simulink model "hpt_1to1_switchlevel"  (R2025a)
settings: Solver=ode23tb  StartTime=0.0  StopTime=0.02  RelTol=1e-3
libraries: spsIGBTLib x19, spsLinearTransformerLib x9, spsGroundLib x4, spsThreePhaseVIMeasurementLib x3, spsSeriesRLCBranchLib x2, spsThreePhaseSeriesRLCBranchLib x2, spsThreePhaseSourceLib x1, spsThreePhaseSeriesRLCLoadLib x1, spsVoltageMeasurementLib x1, spspowerguiLib x1
settings Model: Creator=m1391  LastModifiedBy=m1391

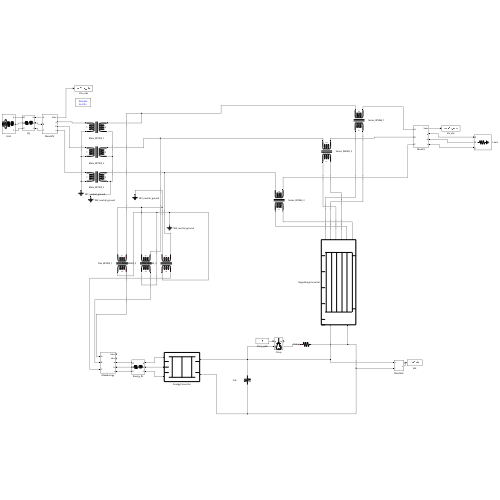
[thumbnail: Simulink's stored preview of the top-level diagram]
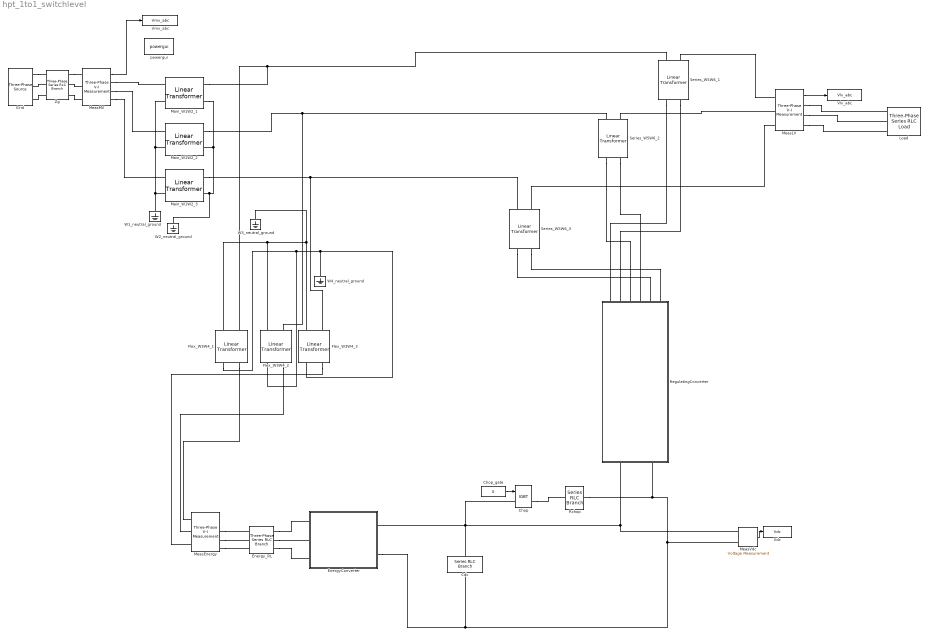
== system hpt_1to1_switchlevel ==
  Cdc : spsSeriesRLCBranchLib/Series RLC Branch  LConnTagsString=__new0  RConnTagsString=__new0  BranchType=C  Resistance=1  Inductance=1e-3  SetiL0=off  InitialCurrent=0  Capacitance=0.0022  Setx0=on  InitialVoltage=800  Measurements=None
  Chop : spsIGBTLib/IGBT  Ron=0.001  Lon=0  Vf=1  Tf=1e-6  Tt=2e-6  IC=0  Rs=1e5  Cs=inf  Measurements=on
  Chop_gate : Constant  Value=0
  EnergyConverter : Subsystem
      mask Display:
      | color('black');
      | plot([10 90 90 10 10],[10 10 90 90 10]);
      | plot([20 80],[78 78]); plot([20 80],[22 22]);
      | plot([28 28],[22 78]); plot([50 50],[22 78]); plot([72 72],[22 78]);
      | plot([10 20],[65 65]); plot([10 20],[50 50]); plot([10 20],[35 35]);
      | plot([80 90],[65 65]); plot([80 90],[35 35]);
  Energy_RL : spsThreePhaseSeriesRLCBranchLib/Three-Phase Series RLC Branch  LConnTagsString=A|B|C  RConnTagsString=A|B|C  BranchType=RL  Resistance=0.05  Inductance=0.003  Capacitance=1e-6  Measurements=None
  Flex_W3W4_1 : spsLinearTransformerLib/Linear Transformer  UNITS=pu  NominalPower=[40000,50]  winding1=[230.9401,0.005,0.02]  winding2=[230.9401,0.005,0.02]  ThreeWindings=off  winding3=[ 315e3 0.002 0.08 ]  RmLm=[ 500 500 ]  Measurements=None  DataType=off
  Flex_W3W4_2 : spsLinearTransformerLib/Linear Transformer  UNITS=pu  NominalPower=[40000,50]  winding1=[230.9401,0.005,0.02]  winding2=[230.9401,0.005,0.02]  ThreeWindings=off  winding3=[ 315e3 0.002 0.08 ]  RmLm=[ 500 500 ]  Measurements=None  DataType=off
  Flex_W3W4_3 : spsLinearTransformerLib/Linear Transformer  UNITS=pu  NominalPower=[40000,50]  winding1=[230.9401,0.005,0.02]  winding2=[230.9401,0.005,0.02]  ThreeWindings=off  winding3=[ 315e3 0.002 0.08 ]  RmLm=[ 500 500 ]  Measurements=None  DataType=off
  Grid : spsThreePhaseSourceLib/Three-Phase Source  InternalConnection=Yg  VoltagePhases=off  Voltage=10000  PhaseAngle=0  Voltage_phases=[25e3 25e3 25e3]/sqrt(3)  PhaseAngles_phases=[0 -120 +120]  Frequency=50  NonIdealSource=on  SpecifyImpedance=off  Resistance=1e-3  Inductance=1e-5  ShortCircuitLevel=100e6  BaseVoltage=25e3  XRratio=7  BusType=swing  Pref=10e3  Qref=0  Prefabc=[10e3, 10e3, 10e3]  Qrefabc=[0, 0, 0]  Qmin=-inf  Qmax=inf
  Load : spsThreePhaseSeriesRLCLoadLib/Three-Phase Series RLC Load  LConnTagsString=A|B|C  Configuration=Y (grounded)  NominalVoltage=400  Vabc=[1e3 1e3 1e3]  Vabcp=[1e3 1e3 1e3]  NominalFrequency=50  UnbalancedPower=off  ActivePower=400000  InductivePower=0  CapacitivePower=0  Pabc=[10e3 9e3 11e3]  QLabc=[100 90 110]  QCabc=[100 90 110]  Pabcp=[10e3 9e3 11e3]  QLabcp=[100 90 110]  QCabcp=[100 90 110]  Measurements=None  LoadType=constant Z
  Main_W1W2_1 : spsLinearTransformerLib/Linear Transformer  UNITS=pu  NominalPower=[133333.3333,50]  winding1=[5773.5027,0.005,0.025]  winding2=[230.9401,0.005,0.025]  ThreeWindings=off  winding3=[ 315e3 0.002 0.08 ]  RmLm=[ 500 500 ]  Measurements=None  DataType=off
  Main_W1W2_2 : spsLinearTransformerLib/Linear Transformer  UNITS=pu  NominalPower=[133333.3333,50]  winding1=[5773.5027,0.005,0.025]  winding2=[230.9401,0.005,0.025]  ThreeWindings=off  winding3=[ 315e3 0.002 0.08 ]  RmLm=[ 500 500 ]  Measurements=None  DataType=off
  Main_W1W2_3 : spsLinearTransformerLib/Linear Transformer  UNITS=pu  NominalPower=[133333.3333,50]  winding1=[5773.5027,0.005,0.025]  winding2=[230.9401,0.005,0.025]  ThreeWindings=off  winding3=[ 315e3 0.002 0.08 ]  RmLm=[ 500 500 ]  Measurements=None  DataType=off
  MeasEnergy : spsThreePhaseVIMeasurementLib/Three-Phase V-I Measurement  VoltageMeasurement=phase-to-ground  SetLabelV=off  LabelV=Vabc  Vpu=off  VpuLL=off  CurrentMeasurement=yes  SetLabelI=off  LabelI=Iabc  Ipu=off  Pbase=100e6  Vbase=500e3  OutputType=Complex  PhasorSimulation=off  PSBequivalent=0
  MeasLV : spsThreePhaseVIMeasurementLib/Three-Phase V-I Measurement  VoltageMeasurement=phase-to-ground  SetLabelV=off  LabelV=Vabc  Vpu=off  VpuLL=off  CurrentMeasurement=no  SetLabelI=off  LabelI=Iabc  Ipu=off  Pbase=100e6  Vbase=500e3  OutputType=Complex  PhasorSimulation=off  PSBequivalent=0
  MeasMV : spsThreePhaseVIMeasurementLib/Three-Phase V-I Measurement  VoltageMeasurement=phase-to-ground  SetLabelV=off  LabelV=Vabc  Vpu=off  VpuLL=off  CurrentMeasurement=no  SetLabelI=off  LabelI=Iabc  Ipu=off  Pbase=100e6  Vbase=500e3  OutputType=Complex  PhasorSimulation=off  PSBequivalent=0
  MeasVdc : spsVoltageMeasurementLib/Voltage Measurement  PhasorSimulation=off  OutputType=Complex  PSBequivalent=0
  Rchop : spsSeriesRLCBranchLib/Series RLC Branch  LConnTagsString=__new0  RConnTagsString=__new0  BranchType=R  Resistance=5.3333  Inductance=1e-3  SetiL0=off  InitialCurrent=0  Capacitance=1e-6  Setx0=off  InitialVoltage=0  Measurements=None
  RegulatingConverter : Subsystem
      mask Display:
      | color('black');
      | plot([5 95 95 5 5],[10 10 90 90 10]);
      | plot([15 85],[78 78]); plot([15 85],[22 22]);
      | plot([18 18],[22 78]); plot([32 32],[22 78]);
      | plot([45 45],[22 78]); plot([59 59],[22 78]);
      | plot([72 72],[22 78]); plot([86 86],[22 78]);
      | plot([5 15],[75 75]); plot([5 15],[60 60]); plot([5 15],[45 45]);
      | plot([5 15],[30 30]); plot([5 15],[15 15]); plot([5 15],[10 10]);
      | plot([85 95],[75 75]); plot([85 95],[25 25]);
  Series_W5W6_1 : spsLinearTransformerLib/Linear Transformer  UNITS=pu  NominalPower=[30000,50]  winding1=[400,0.002,0.03]  winding2=[46.2,0.002,0.03]  ThreeWindings=off  winding3=[ 315e3 0.002 0.08 ]  RmLm=[ 500 500 ]  Measurements=None  DataType=off
  Series_W5W6_2 : spsLinearTransformerLib/Linear Transformer  UNITS=pu  NominalPower=[30000,50]  winding1=[400,0.002,0.03]  winding2=[46.2,0.002,0.03]  ThreeWindings=off  winding3=[ 315e3 0.002 0.08 ]  RmLm=[ 500 500 ]  Measurements=None  DataType=off
  Series_W5W6_3 : spsLinearTransformerLib/Linear Transformer  UNITS=pu  NominalPower=[30000,50]  winding1=[400,0.002,0.03]  winding2=[46.2,0.002,0.03]  ThreeWindings=off  winding3=[ 315e3 0.002 0.08 ]  RmLm=[ 500 500 ]  Measurements=None  DataType=off
  Vdc : ToWorkspace  VariableName=Vdc  SampleTime=2e-05
  Vlv_abc : ToWorkspace  VariableName=Vlv_abc  SampleTime=2e-05
  Vmv_abc : ToWorkspace  VariableName=Vmv_abc  SampleTime=2e-05
  W1_neutral_ground : spsGroundLib/Ground  LConnTagsString=a
  W2_neutral_ground : spsGroundLib/Ground  LConnTagsString=a
  W3_neutral_ground : spsGroundLib/Ground  LConnTagsString=a
  W4_neutral_ground : spsGroundLib/Ground  LConnTagsString=a
  Zg : spsThreePhaseSeriesRLCBranchLib/Three-Phase Series RLC Branch  LConnTagsString=A|B|C  RConnTagsString=A|B|C  BranchType=RL  Resistance=11.7851  Inductance=0.26259  Capacitance=1e-6  Measurements=None
  powergui : spspowerguiLib/powergui  Priority=1  SimulationMode=Discrete  SampleTime=2e-05  frequency=60  Iterations=50  frequencyindice=50  Pbase=100e6  ErrMax=1e-4  UnitsV=kV  UnitsW=MW  buscounter=0  FunctionMessages=off  echomessages=off  EnableUseOfTLC=off  CurrentSourceSwitches=off  DisableSnubberDevices=off  DisableRonSwitches=off  DisableVfSwitches=off  DisplayEquations=off  AutomaticDiscreteSolvers=off  SolverType=Tustin/Backward Euler (TBE)  Interpol=off  ExternalGateDelay=off  methode=off  Ts=100  x0status=blocks  SPID=on  SwTol=0  HookPort=off  NonlinearTolerance=1e-4  nMaxIteration=100  ContinueOnMaxIteration=off  RestoreLinks=warning  ResistiveCurrentMeasurement=off  Frange=[0:2:500]  Ylog=off  Xlog=on  ShowGrid=off  save=off  variable=ZData  structure=0  ZoomFFT=off  StartTime=0.0  cycles=1  DisplayStyle=1  fundamental=60  FreqAxis=off  MaxFrequency=1000  frequencyindicesteady=1  RmsSteady=1  display=off
  wires:
  Chop_gate/1 -> Chop/1
  MeasMV/1 -> Vmv_abc/1
  MeasLV/1 -> Vlv_abc/1
  MeasVdc/1 -> Vdc/1
  connections:
  Grid/RConn1 -- Zg/LConn1
  Zg/RConn1 -- MeasMV/LConn1
  MeasMV/RConn1 -- Main_W1W2_1/LConn1
  Main_W1W2_1/RConn1 -- Series_W5W6_1/RConn1 -- Flex_W3W4_1/LConn1
  Series_W5W6_1/RConn2 -- MeasLV/LConn1
  MeasLV/RConn1 -- Load/LConn1
  Flex_W3W4_1/RConn1 -- MeasEnergy/LConn1
  MeasEnergy/RConn1 -- Energy_RL/LConn1
  Energy_RL/RConn1 -- EnergyConverter/LConn1
  Series_W5W6_1/LConn1 -- RegulatingConverter/LConn1
  Series_W5W6_1/LConn2 -- RegulatingConverter/LConn2
  Grid/RConn2 -- Zg/LConn2
  Zg/RConn2 -- MeasMV/LConn2
  MeasMV/RConn2 -- Main_W1W2_2/LConn1
  Main_W1W2_2/RConn1 -- Series_W5W6_2/RConn1 -- Flex_W3W4_2/LConn1
  Series_W5W6_2/RConn2 -- MeasLV/LConn2
  MeasLV/RConn2 -- Load/LConn2
  Flex_W3W4_2/RConn1 -- MeasEnergy/LConn2
  MeasEnergy/RConn2 -- Energy_RL/LConn2
  Energy_RL/RConn2 -- EnergyConverter/LConn2
  Series_W5W6_2/LConn1 -- RegulatingConverter/LConn3
  Series_W5W6_2/LConn2 -- RegulatingConverter/LConn4
  Grid/RConn3 -- Zg/LConn3
  Zg/RConn3 -- MeasMV/LConn3
  MeasMV/RConn3 -- Main_W1W2_3/LConn1
  Main_W1W2_3/RConn1 -- Series_W5W6_3/RConn1 -- Flex_W3W4_3/LConn1
  Series_W5W6_3/RConn2 -- MeasLV/LConn3
  MeasLV/RConn3 -- Load/LConn3
  Flex_W3W4_3/RConn1 -- MeasEnergy/LConn3
  MeasEnergy/RConn3 -- Energy_RL/LConn3
  Energy_RL/RConn3 -- EnergyConverter/LConn3
  Series_W5W6_3/LConn1 -- RegulatingConverter/LConn5
  Series_W5W6_3/LConn2 -- RegulatingConverter/LConn6
  Main_W1W2_1/LConn2 -- Main_W1W2_2/LConn2 -- Main_W1W2_3/LConn2 -- W1_neutral_ground/LConn1
  Main_W1W2_1/RConn2 -- Main_W1W2_2/RConn2 -- Main_W1W2_3/RConn2 -- W2_neutral_ground/LConn1
  Flex_W3W4_1/LConn2 -- W3_neutral_ground/LConn1 -- Flex_W3W4_3/LConn2 -- Flex_W3W4_2/LConn2
  Flex_W3W4_1/RConn2 -- Flex_W3W4_3/RConn2 -- W4_neutral_ground/LConn1 -- Flex_W3W4_2/RConn2
  MeasVdc/LConn1 -- EnergyConverter/RConn1 -- Cdc/LConn1 -- Chop/LConn1 -- RegulatingConverter/RConn1
  EnergyConverter/RConn2 -- Rchop/RConn1 -- RegulatingConverter/RConn2 -- MeasVdc/LConn2 -- Cdc/RConn1
  Chop/RConn1 -- Rchop/LConn1

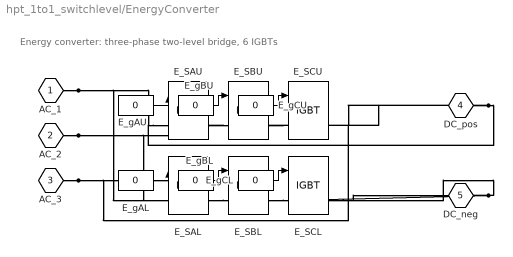
== system hpt_1to1_switchlevel/EnergyConverter ==
  note: Energy converter: three-phase two-level bridge, 6 IGBTs
  E_SAL : spsIGBTLib/IGBT  Ron=0.001  Lon=0  Vf=1  Tf=1e-6  Tt=2e-6  IC=0  Rs=1e5  Cs=inf  Measurements=on
  E_SAU : spsIGBTLib/IGBT  Ron=0.001  Lon=0  Vf=1  Tf=1e-6  Tt=2e-6  IC=0  Rs=1e5  Cs=inf  Measurements=on
  E_SBL : spsIGBTLib/IGBT  Ron=0.001  Lon=0  Vf=1  Tf=1e-6  Tt=2e-6  IC=0  Rs=1e5  Cs=inf  Measurements=on
  E_SBU : spsIGBTLib/IGBT  Ron=0.001  Lon=0  Vf=1  Tf=1e-6  Tt=2e-6  IC=0  Rs=1e5  Cs=inf  Measurements=on
  E_SCL : spsIGBTLib/IGBT  Ron=0.001  Lon=0  Vf=1  Tf=1e-6  Tt=2e-6  IC=0  Rs=1e5  Cs=inf  Measurements=on
  E_SCU : spsIGBTLib/IGBT  Ron=0.001  Lon=0  Vf=1  Tf=1e-6  Tt=2e-6  IC=0  Rs=1e5  Cs=inf  Measurements=on
  E_gAL : Constant  Value=0
  E_gAU : Constant  Value=0
  E_gBL : Constant  Value=0
  E_gBU : Constant  Value=0
  E_gCL : Constant  Value=0
  E_gCU : Constant  Value=0
  AC_1 : PMIOPort  Side=Left
  AC_2 : PMIOPort  Port=2  Side=Left
  AC_3 : PMIOPort  Port=3  Side=Left
  DC_pos : PMIOPort  Port=4  Side=Right
  DC_neg : PMIOPort  Port=5  Side=Right
  wires:
  E_gAU/1 -> E_SAU/1
  E_gAL/1 -> E_SAL/1
  E_gBU/1 -> E_SBU/1
  E_gBL/1 -> E_SBL/1
  E_gCU/1 -> E_SCU/1
  E_gCL/1 -> E_SCL/1
  connections:
  E_SAU/RConn1 -- AC_1/RConn1 -- E_SAL/LConn1
  E_SBU/RConn1 -- AC_2/RConn1 -- E_SBL/LConn1
  E_SCU/RConn1 -- AC_3/RConn1 -- E_SCL/LConn1
  E_SAU/LConn1 -- DC_pos/RConn1 -- E_SBU/LConn1 -- E_SCU/LConn1
  E_SAL/RConn1 -- E_SBL/RConn1 -- DC_neg/RConn1 -- E_SCL/RConn1

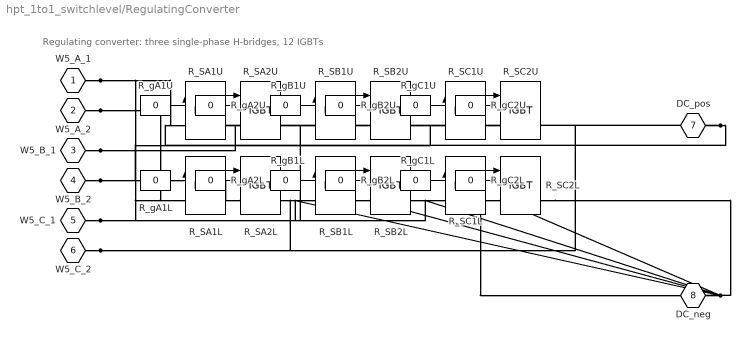
== system hpt_1to1_switchlevel/RegulatingConverter ==
  note: Regulating converter: three single-phase H-bridges, 12 IGBTs
  R_SA1L : spsIGBTLib/IGBT  Ron=0.001  Lon=0  Vf=1  Tf=1e-6  Tt=2e-6  IC=0  Rs=1e5  Cs=inf  Measurements=on
  R_SA1U : spsIGBTLib/IGBT  Ron=0.001  Lon=0  Vf=1  Tf=1e-6  Tt=2e-6  IC=0  Rs=1e5  Cs=inf  Measurements=on
  R_SA2L : spsIGBTLib/IGBT  Ron=0.001  Lon=0  Vf=1  Tf=1e-6  Tt=2e-6  IC=0  Rs=1e5  Cs=inf  Measurements=on
  R_SA2U : spsIGBTLib/IGBT  Ron=0.001  Lon=0  Vf=1  Tf=1e-6  Tt=2e-6  IC=0  Rs=1e5  Cs=inf  Measurements=on
  R_SB1L : spsIGBTLib/IGBT  Ron=0.001  Lon=0  Vf=1  Tf=1e-6  Tt=2e-6  IC=0  Rs=1e5  Cs=inf  Measurements=on
  R_SB1U : spsIGBTLib/IGBT  Ron=0.001  Lon=0  Vf=1  Tf=1e-6  Tt=2e-6  IC=0  Rs=1e5  Cs=inf  Measurements=on
  R_SB2L : spsIGBTLib/IGBT  Ron=0.001  Lon=0  Vf=1  Tf=1e-6  Tt=2e-6  IC=0  Rs=1e5  Cs=inf  Measurements=on
  R_SB2U : spsIGBTLib/IGBT  Ron=0.001  Lon=0  Vf=1  Tf=1e-6  Tt=2e-6  IC=0  Rs=1e5  Cs=inf  Measurements=on
  R_SC1L : spsIGBTLib/IGBT  Ron=0.001  Lon=0  Vf=1  Tf=1e-6  Tt=2e-6  IC=0  Rs=1e5  Cs=inf  Measurements=on
  R_SC1U : spsIGBTLib/IGBT  Ron=0.001  Lon=0  Vf=1  Tf=1e-6  Tt=2e-6  IC=0  Rs=1e5  Cs=inf  Measurements=on
  R_SC2L : spsIGBTLib/IGBT  Ron=0.001  Lon=0  Vf=1  Tf=1e-6  Tt=2e-6  IC=0  Rs=1e5  Cs=inf  Measurements=on
  R_SC2U : spsIGBTLib/IGBT  Ron=0.001  Lon=0  Vf=1  Tf=1e-6  Tt=2e-6  IC=0  Rs=1e5  Cs=inf  Measurements=on
  R_gA1L : Constant  Value=0
  R_gA1U : Constant  Value=0
  R_gA2L : Constant  Value=0
  R_gA2U : Constant  Value=0
  R_gB1L : Constant  Value=0
  R_gB1U : Constant  Value=0
  R_gB2L : Constant  Value=0
  R_gB2U : Constant  Value=0
  R_gC1L : Constant  Value=0
  R_gC1U : Constant  Value=0
  R_gC2L : Constant  Value=0
  R_gC2U : Constant  Value=0
  W5_A_1 : PMIOPort  Side=Left
  W5_A_2 : PMIOPort  Port=2  Side=Left
  W5_B_1 : PMIOPort  Port=3  Side=Left
  W5_B_2 : PMIOPort  Port=4  Side=Left
  W5_C_1 : PMIOPort  Port=5  Side=Left
  W5_C_2 : PMIOPort  Port=6  Side=Left
  DC_pos : PMIOPort  Port=7  Side=Right
  DC_neg : PMIOPort  Port=8  Side=Right
  wires:
  R_gA1U/1 -> R_SA1U/1
  R_gA1L/1 -> R_SA1L/1
  R_gA2U/1 -> R_SA2U/1
  R_gA2L/1 -> R_SA2L/1
  R_gB1U/1 -> R_SB1U/1
  R_gB1L/1 -> R_SB1L/1
  R_gB2U/1 -> R_SB2U/1
  R_gB2L/1 -> R_SB2L/1
  R_gC1U/1 -> R_SC1U/1
  R_gC1L/1 -> R_SC1L/1
  R_gC2U/1 -> R_SC2U/1
  R_gC2L/1 -> R_SC2L/1
  connections:
  R_SA1U/RConn1 -- W5_A_1/RConn1 -- R_SA1L/LConn1
  R_SA2U/RConn1 -- W5_A_2/RConn1 -- R_SA2L/LConn1
  R_SB1U/RConn1 -- W5_B_1/RConn1 -- R_SB1L/LConn1
  R_SB2U/RConn1 -- W5_B_2/RConn1 -- R_SB2L/LConn1
  R_SC1U/RConn1 -- W5_C_1/RConn1 -- R_SC1L/LConn1
  R_SC2U/RConn1 -- W5_C_2/RConn1 -- R_SC2L/LConn1
  R_SA1U/LConn1 -- DC_pos/RConn1 -- R_SA2U/LConn1 -- R_SB1U/LConn1 -- R_SB2U/LConn1 -- R_SC1U/LConn1 -- R_SC2U/LConn1
  R_SA1L/RConn1 -- R_SA2L/RConn1 -- R_SB1L/RConn1 -- R_SB2L/RConn1 -- R_SC1L/RConn1 -- DC_neg/RConn1 -- R_SC2L/RConn1
